simulink model "Simulink_NSR"  (R2016b)
settings: Solver=FixedStepDiscrete  StartTime=0.0  StopTime=10000  FixedStep=1  RelTol=1e-3  EnableMultiTasking=on
libraries: model_library x3
settings Model: NumberOfSteps=200  SnapshotBufferSize=500  SnapshotInterval=100  Creator=dell  LastModifiedBy=dell
settings SolverCC: AutoInsertRateTranBlk=on
settings DataIOCC: LimitDataPoints=on
settings OptimizationCC: LifeSpan=inf
settings DebuggingCC: AllowSymbolicDim=off  SFUnexpectedBacktrackingDiag=warning  SFNoUnconditionalDefaultTransitionDiag=warning  SFExecutionAtInitializationDiag=none
settings GRTTargetCC: TargetLangStandard=C89/C90 (ANSI)
settings ConfigComp: CovMetricSettings=dw  CovHtmlReporting=on  CovSaveCumulativeToWorkspaceVar=on  CovSaveSingleToWorkspaceVar=on  CovShowResultsExplorer=off  CovExternalEMLEnable=off

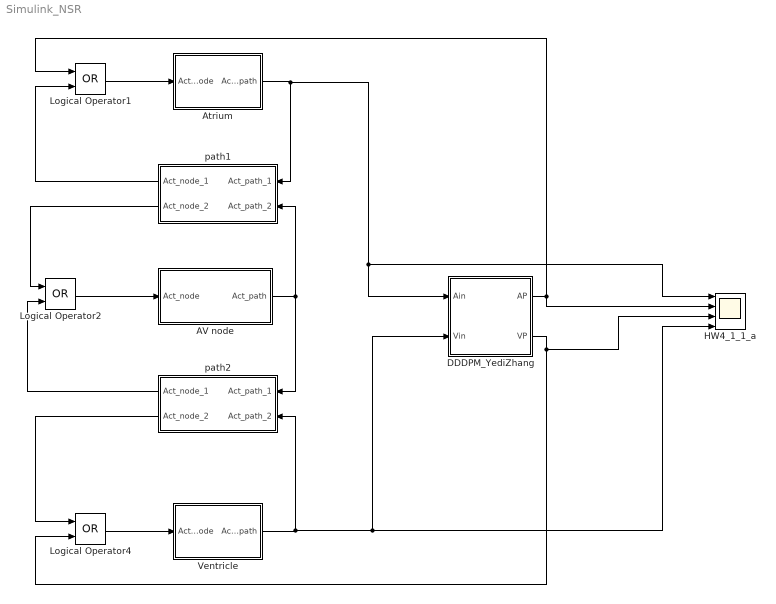
== system Simulink_NSR ==
  "AV node " : Subsystem
  Atrium : Subsystem  AncestorBlock=model_library/Node
  DDDPM_YediZhang : Subsystem
  HW4_1_1_a : Scope  NumInputPorts=4
  Logical Operator1 : Logic  Operator=OR  AllPortsSameDT=off  OutDataTypeStr=boolean
  Logical Operator2 : Logic  Operator=OR  AllPortsSameDT=off  OutDataTypeStr=boolean
  Logical Operator4 : Logic  Operator=OR  AllPortsSameDT=off  OutDataTypeStr=boolean
  Ventricle : Subsystem  AncestorBlock=model_library/Node
  path1 : Subsystem
  path2 : Subsystem
  wires:
  Atrium/1(Act_path) -> HW4_1_1_a/1, DDDPM_YediZhang/1(Ain), path1/1(Act_path_1)
  path1/2(Act_node_2) -> Logical Operator2/1
  Logical Operator2/1 -> "AV node "/1(Act_node)
  "AV node "/1(Act_path) -> path1/2(Act_path_2), path2/1(Act_path_1)
  path2/2(Act_node_2) -> Logical Operator4/1
  Ventricle/1(Act_path) -> DDDPM_YediZhang/2(Vin), HW4_1_1_a/4, path2/2(Act_path_2)
  path2/1(Act_node_1) -> Logical Operator2/2
  path1/1(Act_node_1) -> Logical Operator1/2
  DDDPM_YediZhang/1(AP) -> Logical Operator1/1, HW4_1_1_a/2
  Logical Operator1/1 -> Atrium/1(Act_node)
  DDDPM_YediZhang/2(VP) -> HW4_1_1_a/3, Logical Operator4/2
  Logical Operator4/1 -> Ventricle/1(Act_node)

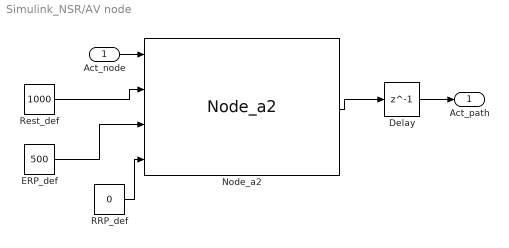
== system Simulink_NSR/AV node  ==
  Act_node : Inport
  Delay : Delay  DelayLength=1  InitialCondition=0
  ERP_def : Constant  Value=500  OutDataTypeStr=uint16
  Node_a2 : model_library/SA-Node/Node_a2
  RRP_def : Constant  Value=0  OutDataTypeStr=uint16
  Rest_def : Constant  Value=1000  OutDataTypeStr=uint16
  Act_path : Outport
  wires:
  Delay/1 -> Act_path/1
  RRP_def/1 -> Node_a2/4
  ERP_def/1 -> Node_a2/3
  Node_a2/1 -> Delay/1
  Act_node/1 -> Node_a2/1
  Rest_def/1 -> Node_a2/2

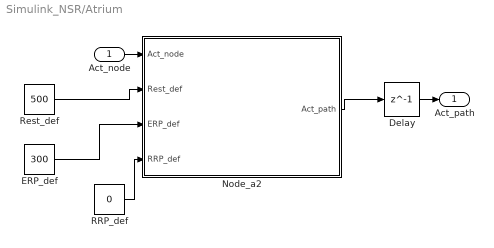
== system Simulink_NSR/Atrium ==
  Act_node : Inport
  Delay : Delay  DelayLength=1  InitialCondition=0
  ERP_def : Constant  Value=300  OutDataTypeStr=uint16
  Node_a2 : Stateflow chart  TreatAsAtomicUnit=on
  RRP_def : Constant  Value=0  OutDataTypeStr=uint16
  Rest_def : Constant  Value=500  OutDataTypeStr=uint16
  Act_path : Outport
  wires:
  Node_a2/1(Act_path) -> Delay/1
  Act_node/1 -> Node_a2/1(Act_node)
  Rest_def/1 -> Node_a2/2(Rest_def)
  ERP_def/1 -> Node_a2/3(ERP_def)
  Delay/1 -> Act_path/1
  RRP_def/1 -> Node_a2/4(RRP_def)

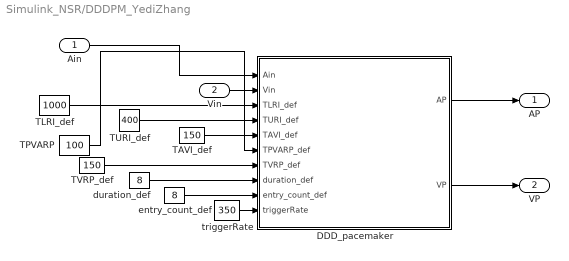
== system Simulink_NSR/DDDPM_YediZhang ==
  Ain : Inport
  Vin : Inport  Port=2
  DDD_pacemaker : Stateflow chart  TreatAsAtomicUnit=on
  TAVI_def : Constant  Value=150  OutDataTypeStr=uint16
  TLRI_def : Constant  Value=1000  OutDataTypeStr=uint16
  TPVARP : Constant  Value=100  OutDataTypeStr=uint16
  TURI_def : Constant  Value=400  OutDataTypeStr=uint16
  TVRP_def : Constant  Value=150  OutDataTypeStr=uint16
  duration_def : Constant  Value=8  OutDataTypeStr=uint16
  entry_count_def : Constant  Value=8  OutDataTypeStr=uint16
  triggerRate : Constant  Value=350  OutDataTypeStr=uint16
  AP : Outport
  VP : Outport  Port=2
  wires:
  DDD_pacemaker/2(VP) -> VP/1
  DDD_pacemaker/1(AP) -> AP/1
  TVRP_def/1 -> DDD_pacemaker/7(TVRP_def)
  Vin/1 -> DDD_pacemaker/2(Vin)
  TPVARP/1 -> DDD_pacemaker/6(TPVARP_def)
  Ain/1 -> DDD_pacemaker/1(Ain)
  TURI_def/1 -> DDD_pacemaker/4(TURI_def)
  TAVI_def/1 -> DDD_pacemaker/5(TAVI_def)
  TLRI_def/1 -> DDD_pacemaker/3(TLRI_def)
  duration_def/1 -> DDD_pacemaker/8(duration_def)
  entry_count_def/1 -> DDD_pacemaker/9(entry_count_def)
  triggerRate/1 -> DDD_pacemaker/10(triggerRate)

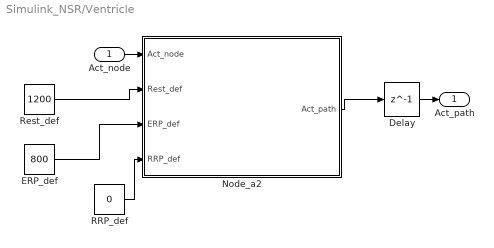
== system Simulink_NSR/Ventricle ==
  Act_node : Inport
  Delay : Delay  DelayLength=1  InitialCondition=0
  ERP_def : Constant  Value=800  OutDataTypeStr=uint16
  Node_a2 : Stateflow chart  TreatAsAtomicUnit=on
  RRP_def : Constant  Value=0  OutDataTypeStr=uint16
  Rest_def : Constant  Value=1200  OutDataTypeStr=uint16
  Act_path : Outport
  wires:
  Node_a2/1(Act_path) -> Delay/1
  Act_node/1 -> Node_a2/1(Act_node)
  Rest_def/1 -> Node_a2/2(Rest_def)
  ERP_def/1 -> Node_a2/3(ERP_def)
  Delay/1 -> Act_path/1
  RRP_def/1 -> Node_a2/4(RRP_def)

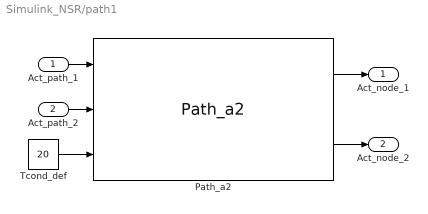
== system Simulink_NSR/path1 ==
  Act_path_1 : Inport
  Act_path_2 : Inport  Port=2
  Path_a2 : model_library/Path/Path_a2
  Tcond_def : Constant  Value=20  OutDataTypeStr=uint16
  Act_node_1 : Outport
  Act_node_2 : Outport  Port=2
  wires:
  Tcond_def/1 -> Path_a2/3
  Act_path_1/1 -> Path_a2/1
  Path_a2/1 -> Act_node_1/1
  Path_a2/2 -> Act_node_2/1
  Act_path_2/1 -> Path_a2/2

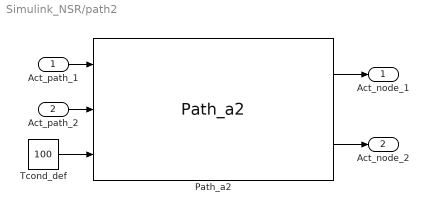
== system Simulink_NSR/path2 ==
  Act_path_1 : Inport
  Act_path_2 : Inport  Port=2
  Path_a2 : model_library/Path/Path_a2
  Tcond_def : Constant  Value=100  OutDataTypeStr=uint16
  Act_node_1 : Outport
  Act_node_2 : Outport  Port=2
  wires:
  Tcond_def/1 -> Path_a2/3
  Act_path_1/1 -> Path_a2/1
  Path_a2/1 -> Act_node_1/1
  Path_a2/2 -> Act_node_2/1
  Act_path_2/1 -> Path_a2/2

== stateflow chart Simulink_NSR/Ventricle/Node_a2 ==
  state node
    settings: description=|
        | temp can be thought of a sub-mode of ERP, which only exists to make sure that act_path is high for one period.
        | 
        | In ERP, if Act_node is received, then it is ignored through that self-transition.
        | 
        | Note this doesn't model variations in cycle length because everytime it is stimulated in RRP, ERP_cur is set to ERP_def again.
    state Rest
    state RRP
    state ERP
    state temp
    (default) -> Rest : {Rest_cur=Rest_def;}
    Rest -> temp [order 3] : [Act_node==false && Rest_cur<=uint16(0)]/{Act_path=true;uptime= uint16(0);ERP_cur=ERP_def;}
    Rest -> temp [order 1] : [Act_node==true]/{Act_path=true;uptime= uint16(0);ERP_cur=ERP_def;}
    Rest -> Rest [order 2] : [Act_node==false && Rest_cur>uint16(0)]/{Rest_cur = Rest_cur - uint16(1);}
    RRP -> Rest [order 1] : [RRP_cur<=0]/{Rest_cur=Rest_def;}
    RRP -> RRP [order 2] : [Act_node==false && RRP_cur>0]/{RRP_cur=RRP_cur-uint16(1);}
    RRP -> temp [order 3] : [Act_node==true]/{Act_path=true;uptime= uint16(0);ERP_cur=ERP_def;}
    ERP -> RRP [order 1] : [ERP_cur<=uint16(0)]/{RRP_cur=RRP_def;}
    temp -> temp [order 1] : [uptime<uint16(1)]/{uptime = uptime + uint16(1);ERP_cur =ERP_cur - uint16(1);}
    temp -> ERP [order 2] : [uptime>=uint16(1)]/{Act_path=false;}
    ERP -> ERP [order 3] : [Act_node==true]
    ERP -> ERP [order 2] : {ERP_cur = ERP_cur - uint16(1);}
  data: Act_node input boolean; Act_path output boolean; Rest_cur local uint16; ERP_cur local uint16; Rest_def input uint16; ERP_def input uint16; uptime local uint16; RRP_cur local uint16; RRP_def input uint16

== stateflow chart Simulink_NSR/DDDPM_YediZhang/DDD_pacemaker ==
  settings: updateMethod=DISCRETE  sampleTime=1
  note: T1
  state DDD_pacemaker
    state PVARP [parallel]
      settings: executionOrder=2
      state PVARP_off
      state AS_up
      note: TP_1
      note: TP_2
      note: TP_3
      state PVARP_on
      note: TP_6
      note: TP_7
      state AR_up
      note: TP_4
      note: TP_5
      (default) -> PVARP_off : {AS=false;}
      PVARP_off -> AS_up [order 1] : [Ain==true]/{AS=true}
      AS_up -> PVARP_off : {AS=false;}
      PVARP_off -> PVARP_on [order 2] : [VS==true || VP_internal==true]/{TPVARP_cur=TPVARP_def;}
      PVARP_on -> PVARP_off [order 3] : [TPVARP_cur<=0]
      AR_up -> PVARP_on : {AR=false,TPVARP_cur=TPVARP_cur-1;}
      PVARP_on -> PVARP_on [order 2] : [TPVARP_cur>0]/
          | {TPVARP_cur = TPVARP_cur - 1;}
      PVARP_on -> AR_up [order 1] : [Ain==true]/{AR=true;}
    state Pre_duration__Counter [parallel]
      settings: executionOrder=6
      note: TPC_3
      state Pre_on
      note: TPC_4
      note: TPC_1
      note: TPC_2
      (default) -> Pre_on : {monitor=false,preCounter=0;}
      Pre_on -> Pre_on [order 2] : [monitor==true&&(AR==true||AS==true)&&TMonitor_cur>triggerRate]/
          | {TMonitor_cur=0, preCounter=preCounter-1;}
      Pre_on -> Pre_on [order 4] : [monitor==true&&(AR==true||AS==true)&&TMonitor_cur<=triggerRate]/{TMonitor_cur=0, preCounter=preCounter+1;}
      Pre_on -> Pre_on [order 1] : [monitor==false&&(AS==true||AR==true)]/{monitor=true,TMonitor_cur=0;}
      Pre_on -> Pre_on [order 3] : [monitor==true&&AR==false&&AS==false]/{TMonitor_cur=TMonitor_cur+1;}
    state VRP [parallel]
      settings: executionOrder=1
      state VRP_off
      state VS_up
      note: TV_1
      note: TV_2
      note: TV_3
      state VRP_on
      note: TV_5
      note: TV_4
      VRP_off -> VS_up [order 1] : [Vin==true]/{VS=true}
      VRP_off -> VRP_on [order 2] : [VP_internal==true]/{TVRP_cur=TVRP_def;}
      VRP_on -> VRP_off [order 2] : [TVRP_cur<=0]
      VS_up -> VRP_on : {TVRP_cur=TVRP_def,VS=false;}
      VRP_on -> VRP_on [order 1] : [TVRP_cur>0]/{TVRP_cur = TVRP_cur - 1;}
    state Duration [parallel]
      settings: executionOrder=7
      state counterMon
      state Dur_on
      note: TD_2
      note: TD_1
      note: TD_4
      note: TD_3
      state VDI_on
      note: TD_6
      note: TD_5
      (default) -> counterMon : {durCounter=0;}
      Dur_on -> Dur_on [order 1] : [VS==true||VP_internal==true]/
          | {durCounter=durCounter+1;}
      counterMon -> Dur_on : [preCounter>=entry_count_def]/
          | {durCounter=0;}
      Dur_on -> counterMon [order 3] : [durCounter>duration_def&&preCounter<=0]/
          | {ifSwitch=false;}
      VDI_on -> counterMon [order 1] : [preCounter<=0]/{ifSwitch=false,durCounter=0;}
      Dur_on -> VDI_on [order 2] : [durCounter>duration_def&&preCounter>0]/{ifSwitch=true;}
      VDI_on -> VDI_on [order 2] : [preCounter>0]
    state LRI [parallel]
      settings: executionOrder=5
      note: TL_8
      note: TL_5
      state LRI_off
      state LRI_wait
      note: TL_2
      note: TL_3
      note: TL_7
      note: TL_4
      note: TL_6
      note: TL_9
      state LRI_VP_up
      note: TL_1
      note: TL_11
      note: TL_12
      note: TL_14
      note: TL_16
      state SM_LRI
      note: TL_10
      note: TL_15
      note: TL_13
      (default) -> LRI_off : {TLRI_cur = TLRI_def,AP_up=2,AP=false,AP_internal=false;}
      LRI_wait -> LRI_wait [order 3] : [ifSwitch==false&&TLRI_cur>0]
          | /{TLRI_cur=TLRI_cur-1;}
      LRI_off -> LRI_wait [order 5] : [ifSwitch==false&&TLRI_cur<=(TAVI_def)]/
          | {AP=true,AP_up=1,AP_internal=true,TLRI_cur = TLRI_cur-1;}
      LRI_off -> LRI_off [order 2] : [ifSwitch==false &&(VS==true||VP_internal==true)]/
          | {TLRI_cur=TLRI_def;}
      LRI_off -> LRI_wait [order 3] : [ifSwitch==false&&AS==true]/{TLRI_cur = TLRI_cur-1;}
      LRI_wait -> LRI_off [order 2] : [ifSwitch==false&&(VS==true||VP_internal==true)]/{TLRI_cur=TLRI_def;}
      LRI_wait -> SM_LRI [order 5] : [ifSwitch==true]
      LRI_wait -> LRI_VP_up [order 4] : [ifSwitch==false&&TLRI_cur<=0]/
          | {VP=true,VP_internal=true;}
      LRI_wait -> LRI_wait [order 1] : [AP_up==1]/
          | {AP_up=AP_up+1,AP=false,AP_internal=false,
          | TLRI_cur=TLRI_cur-1;}
      LRI_off -> SM_LRI [order 1] : [ifSwitch==true]/{TLRI_cur = TLRI_cur-1;}
      LRI_VP_up -> LRI_off [order 1] : [ifSwitch==false]/
          | {VP=false, VP_internal=false, TLRI_cur=TLRI_def;}
      LRI_off -> LRI_off [order 4] : [ifSwitch==false&&TLRI_cur>(TAVI_def)]/
          | {TLRI_cur = TLRI_cur-1;}
      SM_LRI -> LRI_off [order 4] : [ifSwitch==false]/{TLRI_cur = TLRI_cur-1;}
      SM_LRI -> LRI_VP_up [order 2] : [ifSwitch==true&&TLRI_cur<=0]/{VP=true,VP_internal=true;}
      LRI_VP_up -> SM_LRI [order 2] : [ifSwitch==true]/{VP=false,VP_internal=false,TLRI_cur=TLRI_def;}
      SM_LRI -> SM_LRI [order 3] : [ifSwitch==true&&TLRI_cur>0]/
          | {TLRI_cur=TLRI_cur-1;}
      SM_LRI -> SM_LRI [order 1] : [ifSwitch==true&&VS==true]/{TLRI_cur=TLRI_def;}
    state AVI [parallel]
      settings: executionOrder=4
      state AVI_off
      state AVI_on
      note: TA_2
      note: TA_4
      note: TA_1
      note: TA_3
      note: TA_6
      state AVI_VP_up
      note: TA_5
      note: TA_7
      (default) -> AVI_off : {VP=false,VP_internal=false;}
      AVI_off -> AVI_off [order 2] : [ifSwitch==true]
      AVI_on -> AVI_on [order 3] : [ifSwitch==false&&TAVI_cur>0]/{TAVI_cur=TAVI_cur-1;}
      AVI_off -> AVI_on [order 1] : [ifSwitch==false &&(AP_internal==true || AS==true)]/
          | {TAVI_cur=TAVI_def;}
      AVI_on -> AVI_off [order 2] : [VS==true||VP_internal==true||ifSwitch==true]
      AVI_VP_up -> AVI_off : {VP=false,VP_internal=false;}
      AVI_on -> AVI_VP_up [order 1] : [ifSwitch==false&&TAVI_cur<=0&&URI_block==false]/
          | {VP=true, VP_internal=true;}
      AVI_on -> AVI_on [order 4] : [ifSwitch==false&&TAVI_cur<=0 && URI_block==true]
    state URI [parallel]
      settings: executionOrder=3
      note: TU_2
      state URI_off
      state URI_on
      note: TU_1
      note: TU_4
      note: TU_3
      (default) -> URI_off : {URI_block=false;}
      URI_on -> URI_on [order 1] : [VS==true || VP_internal==true]/
          | {TURI_cur=TURI_def, URI_block=true;}
      URI_off -> URI_on : [VS==true || VP_internal==true]/
          | {TURI_cur=TURI_def, URI_block=true;}
      URI_on -> URI_off [order 3] : [TURI_cur<=0]/{URI_block=false;}
      URI_on -> URI_on [order 2] : [TURI_cur>0]/{TURI_cur = TURI_cur - 1;}
    (default) -> VRP_off : {VS=false}
  (default) -> DDD_pacemaker : {ifSwitch=false, VS=false, VP_internal=false, VP=false, AS=false,AR=false,AP_internal=false,  AP_up=2,  AP=false, preCounter=0, URI_block=false, TVRP_cur=TVRP_def, TPVARP_cur = TPVARP_def, TAVI_cur = TAVI_def, TLRI_cur = TLRI_def, TURI_cur = TURI_def;}
  data: Ain input; VS local; Vin input; AP output; VP output; TVRP_cur local; AS local; TPVARP_cur local; TAVI_cur local; URI_block local; TLRI_cur local; TURI_cur local; AP_up local; VP_internal local; AP_internal local; TLRI_def input uint16; TURI_def input uint16; TAVI_def input uint16; TPVARP_def input uint16; TVRP_def input uint16 =150; ifSwitch local; AR local; TMonitor_cur local; durCounter local; monitor local; duration_def input uint16 =8; entry_count_def input uint16 =8; triggerRate input uint16; preCounter local

== stateflow chart Simulink_NSR/Atrium/Node_a2 ==
  state node
    settings: description=|
        | temp can be thought of a sub-mode of ERP, which only exists to make sure that act_path is high for one period.
        | 
        | In ERP, if Act_node is received, then it is ignored through that self-transition.
        | 
        | Note this doesn't model variations in cycle length because everytime it is stimulated in RRP, ERP_cur is set to ERP_def again.
    state Rest
    state RRP
    state ERP
    state temp
    (default) -> Rest : {Rest_cur=Rest_def;}
    Rest -> temp [order 3] : [Act_node==false && Rest_cur<=uint16(0)]/{Act_path=true;uptime= uint16(0);ERP_cur=ERP_def;}
    Rest -> temp [order 1] : [Act_node==true]/{Act_path=true;uptime= uint16(0);ERP_cur=ERP_def;}
    Rest -> Rest [order 2] : [Act_node==false && Rest_cur>uint16(0)]/{Rest_cur = Rest_cur - uint16(1);}
    RRP -> Rest [order 1] : [RRP_cur<=0]/{Rest_cur=Rest_def;}
    RRP -> RRP [order 2] : [Act_node==false && RRP_cur>0]/{RRP_cur=RRP_cur-uint16(1);}
    RRP -> temp [order 3] : [Act_node==true]/{Act_path=true;uptime= uint16(0);ERP_cur=ERP_def;}
    ERP -> RRP [order 1] : [ERP_cur<=uint16(0)]/{RRP_cur=RRP_def;}
    temp -> temp [order 1] : [uptime<uint16(1)]/{uptime = uptime + uint16(1);ERP_cur =ERP_cur - uint16(1);}
    temp -> ERP [order 2] : [uptime>=uint16(1)]/{Act_path=false;}
    ERP -> ERP [order 3] : [Act_node==true]
    ERP -> ERP [order 2] : {ERP_cur = ERP_cur - uint16(1);}
  data: Act_node input boolean; Act_path output boolean; Rest_cur local uint16; ERP_cur local uint16; Rest_def input uint16; ERP_def input uint16; uptime local uint16; RRP_cur local uint16; RRP_def input uint16
